simulink model "top_model"  (R2025b)
settings: Solver=FixedStepDiscrete  StartTime=0.0  StopTime=t_stop  FixedStep=Ts_plant  RelTol=1e-3
undefined symbols (not defined in the file): c_d, c_rr, DiscIntNeverNeededParam, F_brake_max, F_drive_max, Kp_brake, Kp_speed, Kp_steer, m, tau_steer, Ts_can, Ts_ctrl, Ts_plant
settings Model: Creator=jahnaviveeraboyini  LastModifiedBy=jahnaviveeraboyini

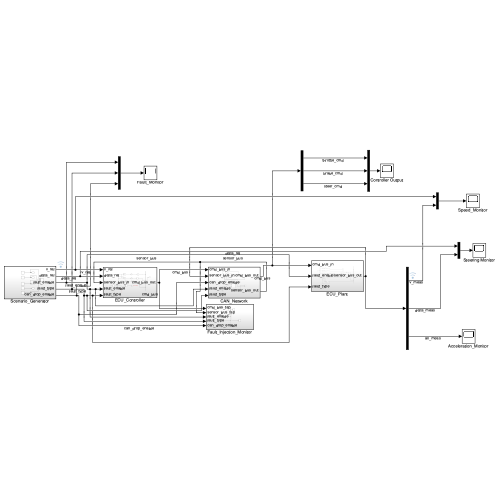
[thumbnail: Simulink's stored preview of the top-level diagram]
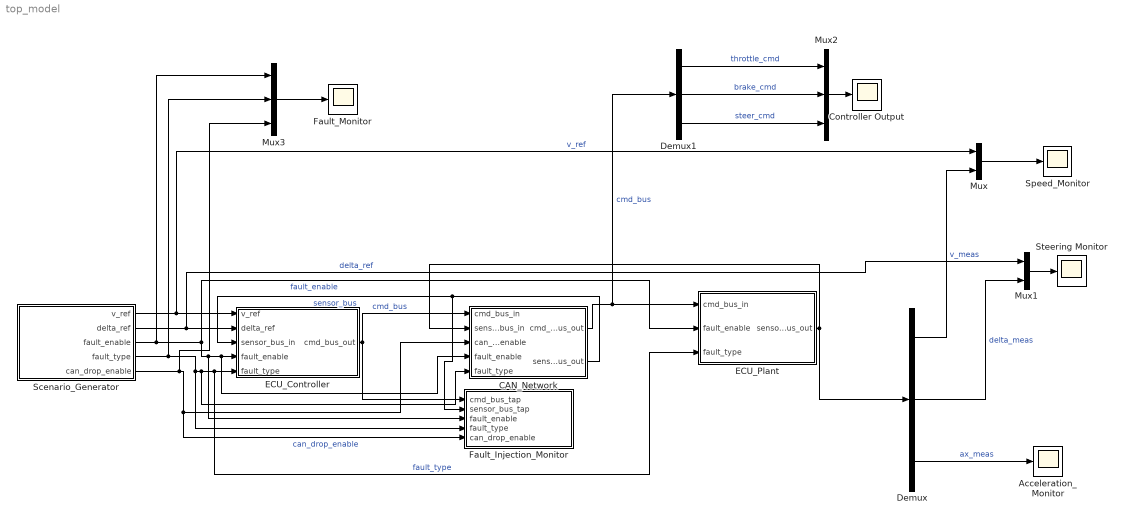
== system top_model ==
  Acceleration_Monitor : Scope
      settings: ActiveDisplayYMinimum=-0.71398527983090265  ActiveDisplayYMaximum=0.071924290351581752  DataLoggingVariableName=ScopeData7
  CAN_Network : Subsystem
  Controller Output : Scope
      settings: ActiveDisplayYMinimum=-0.12499999999999997  ActiveDisplayYMaximum=1.125  DataLoggingVariableName=ScopeData8
  Demux : Demux  Outputs=3
  Demux1 : Demux  Outputs=3
  ECU_Controller : Subsystem
  ECU_Plant : Subsystem
  Fault_Injection_Monitor : Subsystem
  Fault_Monitor : Scope
      settings: ActiveDisplayYMinimum=-0.12499999999999997  ActiveDisplayYMaximum=1.125  DataLoggingVariableName=ScopeData9
  Mux : Mux  Inputs=2
  Mux1 : Mux  Inputs=2
  Mux2 : Mux  Inputs=3
  Mux3 : Mux  Inputs=3
  Scenario_Generator : Subsystem
  Speed_Monitor : Scope
      settings: ActiveDisplayYMinimum=-30.08374757605813  ActiveDisplayYMaximum=20.009305286228681  DataLoggingVariableName=ScopeData5
  Steering Monitor : Scope
      settings: ActiveDisplayYMinimum=-1.2499999999999998  ActiveDisplayYMaximum=11.25  DataLoggingVariableName=ScopeData6
  wires:
  Scenario_Generator/1(v_ref) -> Mux/1, ECU_Controller/1(v_ref)  "v_ref"
  Scenario_Generator/2(delta_ref) -> Mux1/1, ECU_Controller/2(delta_ref)  "delta_ref"
  Scenario_Generator/3(fault_enable) -> Mux3/1, CAN_Network/4(fault_enable), ECU_Controller/4(fault_enable), Fault_Injection_Monitor/3(fault_enable), ECU_Plant/2(fault_enable)  "fault_enable"
  Scenario_Generator/4(fault_type) -> Mux3/2, ECU_Plant/3(fault_type), ECU_Controller/5(fault_type), CAN_Network/5(fault_type), Fault_Injection_Monitor/4(fault_type)  "fault_type"
  Scenario_Generator/5(can_drop_enable) -> Mux3/3, Fault_Injection_Monitor/5(can_drop_enable), CAN_Network/3(can_drop_enable)  "can_drop_enable"
  ECU_Controller/1(cmd_bus_out) -> Fault_Injection_Monitor/1(cmd_bus_tap), CAN_Network/1(cmd_bus_in)  "cmd_bus"
  CAN_Network/2(sensor_bus_out) -> Fault_Injection_Monitor/2(sensor_bus_tap), ECU_Controller/3("sensor_bus_in ")  "sensor_bus"
  CAN_Network/1(cmd_bus_out) -> Demux1/1, ECU_Plant/1(cmd_bus_in)  "cmd_bus"
  ECU_Plant/1(sensor_bus_out) -> CAN_Network/2(sensor_bus_in), Demux/1
  Demux/1 -> Mux/2  "v_meas"
  Demux/2 -> Mux1/2  "delta_meas"
  Demux/3 -> Acceleration_Monitor/1  "ax_meas"
  Mux/1 -> Speed_Monitor/1
  Mux1/1 -> Steering Monitor/1
  Demux1/1 -> Mux2/1  "throttle_cmd"
  Demux1/2 -> Mux2/2  "brake_cmd"
  Demux1/3 -> Mux2/3  "steer_cmd"
  Mux2/1 -> Controller Output/1
  Mux3/1 -> Fault_Monitor/1

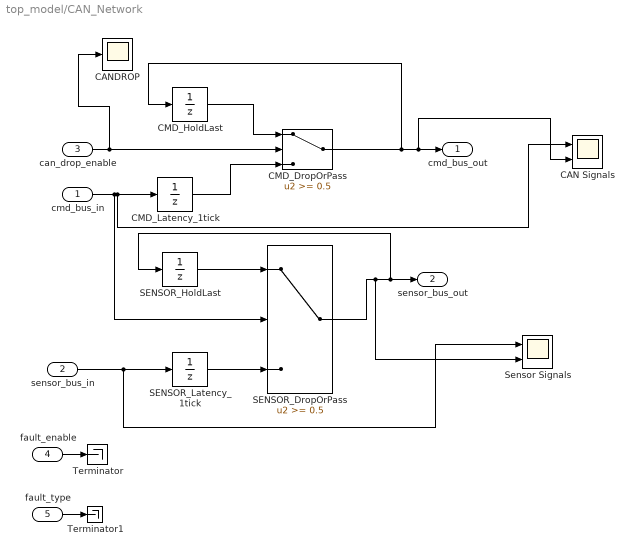
== system top_model/CAN_Network ==
  cmd_bus_in : Inport
  sensor_bus_in : Inport  Port=2
  can_drop_enable : Inport  Port=3
  fault_enable : Inport  Port=4
  fault_type : Inport  Port=5
  CAN Signals : Scope  NumInputPorts=2
      settings: ActiveDisplayYMinimum=-1  ActiveDisplayYMaximum=1
  CANDROP : Scope
      settings: ActiveDisplayYMinimum=-0.12499999999999997  ActiveDisplayYMaximum=1.125  DataLoggingVariableName=ScopeData3
  CMD_DropOrPass : Switch  Threshold=0.5  SaturateOnIntegerOverflow=off  InputSameDT=off
  CMD_HoldLast : UnitDelay  SampleTime=-1  HasFrameUpgradeWarning=on
  CMD_Latency_1tick : UnitDelay  SampleTime=Ts_can  HasFrameUpgradeWarning=on
  SENSOR_DropOrPass : Switch  Threshold=0.5  SaturateOnIntegerOverflow=off  InputSameDT=off
  SENSOR_HoldLast : UnitDelay  SampleTime=-1  HasFrameUpgradeWarning=on
  SENSOR_Latency_1tick : UnitDelay  SampleTime=Ts_can  HasFrameUpgradeWarning=on
  Sensor Signals : Scope  NumInputPorts=2
      settings: ActiveDisplayYMinimum=-1  ActiveDisplayYMaximum=1  DataLoggingVariableName=ScopeData2
  Terminator : Terminator
  Terminator1 : Terminator
  cmd_bus_out : Outport
  sensor_bus_out : Outport  Port=2
  wires:
  cmd_bus_in/1 -> SENSOR_DropOrPass/2, CAN Signals/1, CMD_Latency_1tick/1
  sensor_bus_in/1 -> Sensor Signals/1, SENSOR_Latency_1tick/1
  can_drop_enable/1 -> CANDROP/1, CMD_DropOrPass/2
  CMD_HoldLast/1 -> CMD_DropOrPass/1
  CMD_Latency_1tick/1 -> CMD_DropOrPass/3
  CMD_DropOrPass/1 -> CMD_HoldLast/1, CAN Signals/2, cmd_bus_out/1
  SENSOR_Latency_1tick/1 -> SENSOR_DropOrPass/3
  SENSOR_HoldLast/1 -> SENSOR_DropOrPass/1
  SENSOR_DropOrPass/1 -> Sensor Signals/2, SENSOR_HoldLast/1, sensor_bus_out/1
  fault_enable/1 -> Terminator/1
  fault_type/1 -> Terminator1/1

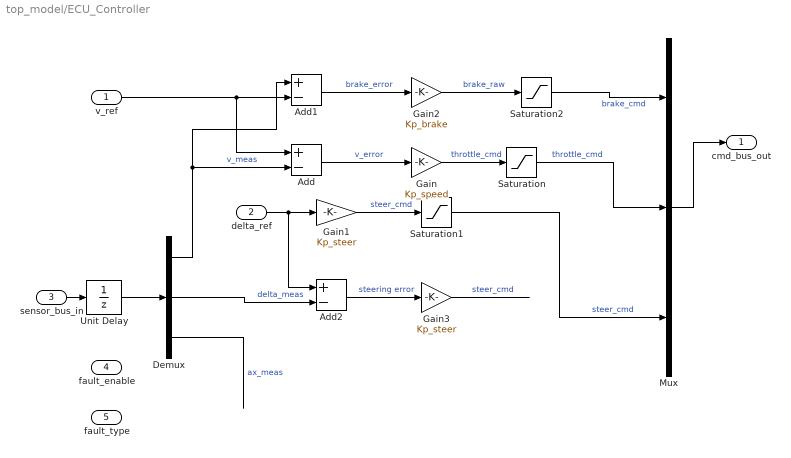
== system top_model/ECU_Controller ==
  v_ref : Inport
  delta_ref : Inport  Port=2
  "sensor_bus_in " : Inport  Port=3
  fault_enable : Inport  Port=4
  fault_type : Inport  Port=5
  Add : Sum  Inputs=+-
  Add1 : Sum  Inputs=+-
  Add2 : Sum  Inputs=+-
  Demux : Demux  Outputs=3
  Gain : Gain  Gain=Kp_speed
  Gain1 : Gain  Gain=Kp_steer
  Gain2 : Gain  Gain=Kp_brake
  Gain3 : Gain  Gain=Kp_steer
  Mux : Mux  Inputs=3
  Saturation : Saturate  UpperLimit=1  LowerLimit=0
  Saturation1 : Saturate  UpperLimit=1  LowerLimit=-1
  Saturation2 : Saturate  UpperLimit=1  LowerLimit=0
  Unit Delay : UnitDelay  SampleTime=Ts_ctrl  HasFrameUpgradeWarning=on
  cmd_bus_out : Outport
  wires:
  Demux/1 -> Add1/1, Add/2  "v_meas"
  Demux/2 -> Add2/2  "delta_meas"
  Demux/3 -> ?  "ax_meas"
  v_ref/1 -> Add1/2, Add/1
  Add/1 -> Gain/1  "v_error"
  Gain/1 -> Saturation/1  "throttle_cmd"
  Saturation/1 -> Mux/2  "throttle_cmd"
  delta_ref/1 -> Add2/1, Gain1/1
  Gain1/1 -> Saturation1/1  "steer_cmd"
  Saturation1/1 -> Mux/3  "steer_cmd"
  Add1/1 -> Gain2/1  "brake_error"
  Gain2/1 -> Saturation2/1  "brake_raw"
  Saturation2/1 -> Mux/1  "brake_cmd"
  Add2/1 -> Gain3/1  "steering error"
  Gain3/1 -> ?  "steer_cmd"
  Mux/1 -> cmd_bus_out/1
  "sensor_bus_in "/1 -> Unit Delay/1
  Unit Delay/1 -> Demux/1

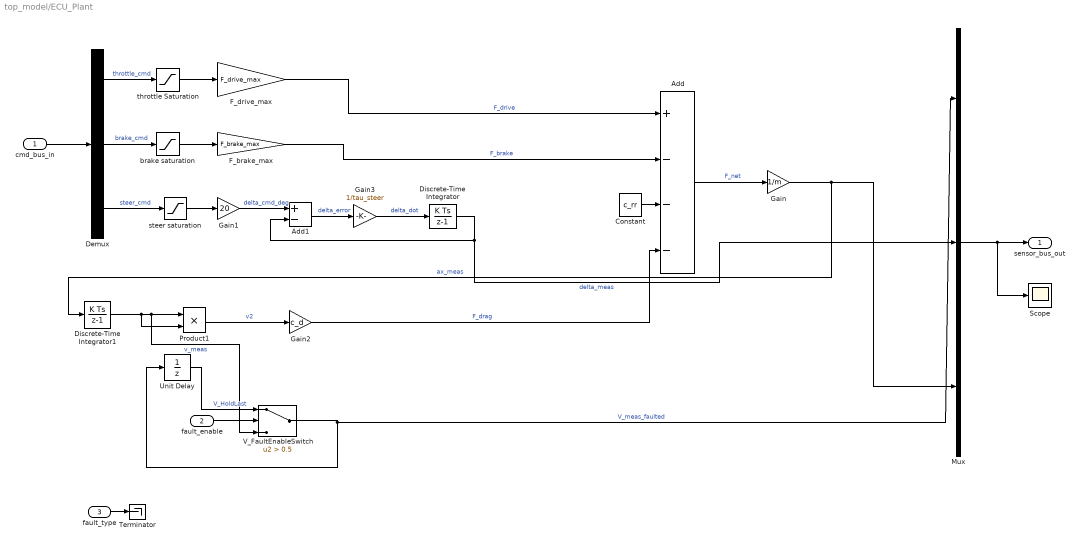
== system top_model/ECU_Plant ==
  cmd_bus_in : Inport
  fault_enable : Inport  Port=2
  fault_type : Inport  Port=3
  Add : Sum  Inputs=+---
  Add1 : Sum  Inputs=+-
  Constant : Constant  Value=c_rr
  Demux : Demux  Outputs=3
  Discrete-Time Integrator : DiscreteIntegrator  SampleTime=-1  ICPrevOutput=DiscIntNeverNeededParam  ICPrevScaledInput=DiscIntNeverNeededParam
  Discrete-Time Integrator1 : DiscreteIntegrator  SampleTime=Ts_plant  ICPrevOutput=DiscIntNeverNeededParam  ICPrevScaledInput=DiscIntNeverNeededParam
  F_brake_max : Gain  Gain=F_brake_max
  F_drive_max : Gain  Gain=F_drive_max
  Gain : Gain  Gain=1/m
  Gain1 : Gain  Gain=20
  Gain2 : Gain  Gain=c_d
  Gain3 : Gain  Gain=1/tau_steer
  Mux : Mux  Inputs=3
  Product1 : Product
  Scope : Scope
      settings: ActiveDisplayYMinimum=-30.70874757605813  ActiveDisplayYMaximum=25.634305286228681  DataLoggingVariableName=ScopeData4
  Terminator : Terminator
  Unit Delay : UnitDelay  SampleTime=-1  HasFrameUpgradeWarning=on
  V_FaultEnableSwitch : Switch  Criteria=u2 > Threshold  Threshold=0.5  SaturateOnIntegerOverflow=off  InputSameDT=off
  brake saturation : Saturate  UpperLimit=1  LowerLimit=0
  steer saturation : Saturate  UpperLimit=1  LowerLimit=-1
  throttle Saturation : Saturate  UpperLimit=1  LowerLimit=0
  sensor_bus_out : Outport
  wires:
  cmd_bus_in/1 -> Demux/1
  Demux/3 -> steer saturation/1  "steer_cmd"
  Demux/2 -> brake saturation/1  "brake_cmd"
  Demux/1 -> throttle Saturation/1  "throttle_cmd"
  throttle Saturation/1 -> F_drive_max/1
  brake saturation/1 -> F_brake_max/1
  F_drive_max/1 -> Add/1  "F_drive"
  F_brake_max/1 -> Add/2  "F_brake"
  Constant/1 -> Add/3
  Gain2/1 -> Add/4  "F_drag"
  Product1/1 -> Gain2/1  "v2"
  Discrete-Time Integrator1/1 -> Product1/1, V_FaultEnableSwitch/3, Product1/2  "v_meas"
  Add/1 -> Gain/1  "F_net"
  Gain/1 -> Discrete-Time Integrator1/1, Mux/3  "ax_meas"
  steer saturation/1 -> Gain1/1
  Gain1/1 -> Add1/1  "delta_cmd_deg"
  Add1/1 -> Gain3/1  "delta_error"
  Gain3/1 -> Discrete-Time Integrator/1  "delta_dot"
  Discrete-Time Integrator/1 -> Mux/2, Add1/2  "delta_meas"
  fault_enable/1 -> V_FaultEnableSwitch/2
  Unit Delay/1 -> V_FaultEnableSwitch/1  "V_HoldLast"
  Mux/1 -> Scope/1, sensor_bus_out/1
  V_FaultEnableSwitch/1 -> Mux/1, Unit Delay/1  "V_meas_faulted"
  fault_type/1 -> Terminator/1

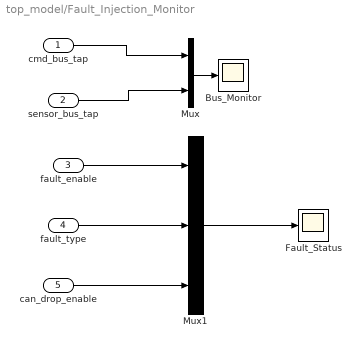
== system top_model/Fault_Injection_Monitor ==
  cmd_bus_tap : Inport
  sensor_bus_tap : Inport  Port=2
  fault_enable : Inport  Port=3
  fault_type : Inport  Port=4
  can_drop_enable : Inport  Port=5
  Bus_Monitor : Scope
      settings: DataLoggingVariableName=ScopeData11
  Fault_Status : Scope
      settings: DataLoggingVariableName=ScopeData10
  Mux : Mux  Inputs=2
  Mux1 : Mux  Inputs=3
  wires:
  fault_enable/1 -> Mux1/1
  fault_type/1 -> Mux1/2
  can_drop_enable/1 -> Mux1/3
  Mux1/1 -> Fault_Status/1
  cmd_bus_tap/1 -> Mux/1
  sensor_bus_tap/1 -> Mux/2
  Mux/1 -> Bus_Monitor/1

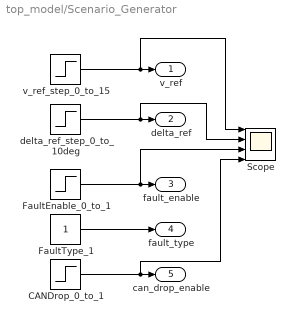
== system top_model/Scenario_Generator ==
  CANDrop_0_to_1 : Step  Time=12  SampleTime=0
  FaultEnable_0_to_1 : Step  Time=10  SampleTime=0
  FaultType_1 : Constant
  Scope : Scope  NumInputPorts=4
      settings: ActiveDisplayYMinimum=-1.8749999999999996  ActiveDisplayYMaximum=16.875
  delta_ref_step_0_to_10deg : Step  Time=6  After=10  SampleTime=0
  v_ref_step_0_to_15 : Step  Time=2  After=15  SampleTime=0
  v_ref : Outport
  delta_ref : Outport  Port=2
  fault_enable : Outport  Port=3
  fault_type : Outport  Port=4
  can_drop_enable : Outport  Port=5
  wires:
  FaultType_1/1 -> fault_type/1
  CANDrop_0_to_1/1 -> Scope/4, can_drop_enable/1
  v_ref_step_0_to_15/1 -> Scope/1, v_ref/1
  delta_ref_step_0_to_10deg/1 -> Scope/2, delta_ref/1
  FaultEnable_0_to_1/1 -> Scope/3, fault_enable/1
